simulink model "vrednotenje"  (R2020b)
settings: Solver=ode45  StartTime=0.0  StopTime=Tkon  RelTol=1e-3  EnableMultiTasking=on
values from neighbouring files (symbols this model uses):
  Ts = 0.01    [signali.mat]
settings Model: Creator=Administrator  LastModifiedBy=Acer
settings DataIOCC: LimitDataPoints=on  SaveFormat=Array  ReturnWorkspaceOutputs=off
settings OptimizationCC: LifeSpan=inf
settings DebuggingCC: SolverPrmCheckMsg=warning  SFUnexpectedBacktrackingDiag=warning  SFNoUnconditionalDefaultTransitionDiag=warning  SFExecutionAtInitializationDiag=none  ArithmeticOperatorsInVariantConditions=warning
settings HardwareCC: ProdBitPerPointer=32  ProdBitPerSizeT=32  ProdBitPerPtrDiffT=32  ProdLargestAtomicFloat=None  ProdIntDivRoundTo=Undefined  ProdEndianess=Unspecified  ProdWordSize=32  ProdHWDeviceType=32-bit Generic
settings ModelReferenceCC: PropagateSignalLabelsOutOfModel=off
settings SFSimCC: SimUseLocalCustomCode=off  CustomCodeUndefinedFunction=UseInterfaceOnly
settings RTWCC: RTWUseLocalCustomCode=off
settings CodeAppCC: StateflowObjectComments=on
settings GRTTargetCC: TargetLangStandard=C89/C90 (ANSI)
settings ConfigComp: CovMetricSettings=dw  CovSaveCumulativeToWorkspaceVar=on  CovSaveSingleToWorkspaceVar=on  CovExternalEMLEnable=off  CovSFcnEnable=off

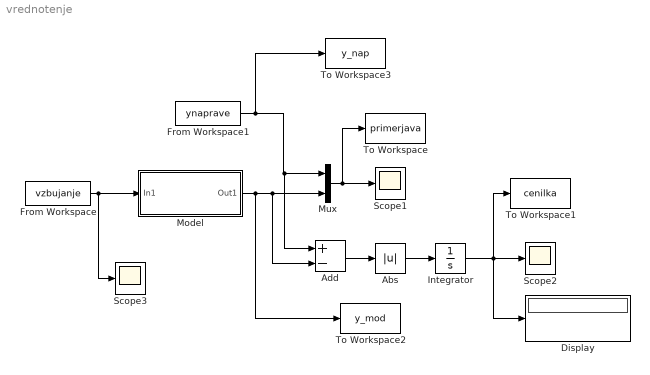
== system vrednotenje ==
  Abs : Abs
  Add : Sum  Inputs=+-
  Display : Display
  From Workspace : FromWorkspace  VariableName=vzbujanje
  From Workspace1 : FromWorkspace  VariableName=ynaprave  SampleTime=Ts
  Integrator : Integrator
  Model : Subsystem
  Mux : Mux  Inputs=2
  Scope1 : Scope
  Scope2 : Scope
  Scope3 : Scope
  To Workspace : ToWorkspace  VariableName=primerjava  SaveFormat=Timeseries  SampleTime=-1
  To Workspace1 : ToWorkspace  VariableName=cenilka  SaveFormat=Timeseries  SampleTime=-1
  To Workspace2 : ToWorkspace  VariableName=y_mod  SampleTime=Ts
  To Workspace3 : ToWorkspace  VariableName=y_nap  SampleTime=Ts
  wires:
  Mux/1 -> To Workspace/1, Scope1/1
  Add/1 -> Abs/1
  Abs/1 -> Integrator/1
  Integrator/1 -> To Workspace1/1, Display/1, Scope2/1
  From Workspace/1 -> Scope3/1, Model/1(In1)
  From Workspace1/1 -> To Workspace3/1, Add/1, Mux/1
  Model/1(Out1) -> To Workspace2/1, Add/2, Mux/2

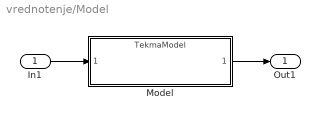
== system vrednotenje/Model ==
  In1 : Inport
  Model : ModelReference  ModelNameDialog=TekmaModel.slx  SimulationMode=Normal  ModelReferenceVersion=1.79
  Out1 : Outport
  wires:
  In1/1 -> Model/1
  Model/1 -> Out1/1
